simulink model "MotorIPMSVC"  (R2023a)
settings: Solver=FixedStepDiscrete  StartTime=0.0  StopTime=10.0  FixedStep=0.0001  RelTol=1e-3
InitFcn:
  | svc_go_init;
model workspace (MATLAB code in the model file):
  | cmdLim = Simulink.Parameter;
  | cmdLim.Value = 15;
  | cmdLim.Description = 'Limit for controlling the maximum surface command angle.';
  | cmdLim.Min = 0;
  | cmdLim.Max = 90;
  | cmdLim.DocUnits = 'deg';
  | 
  | dispGain = Simulink.Parameter;
  | dispGain.Value = 0.75;
  | dispGain.Description = 'Gain applied to the displacement error.';
  | dispGain.Min = 0;
  | dispGain.Max = [];
  | dispGain.DocUnits = 'deg/sec/deg';
  | 
  | dispLim = Simulink.Parameter;
  | dispLim.Value = 30;
  | dispLim.Description = 'Limit for controlling the maximum commanded angle.';
  | dispLim.Min = 0;
  | dispLim.Max = 180;
  | dispLim.DocUnits = 'deg';
  | 
  | intGain = Simulink.Parameter;
  | intGain.Value = 0.5;
  | intGain.Description = 'Gain applied to the integral error.';
  | intGain.Min = 0;
  | intGain.Max = [];
  | intGain.DocUnits = 'deg/sec/deg/sec';
  | 
  | intLim = Simulink.Parameter;
  | intLim.Value = 5;
  | intLim.Description = 'Limit for controlling the maximum commanded angle.';
  | intLim.Min = 0;
  | intLim.Max = 90;
  | intLim.DocUnits = 'deg';
  | 
  | rateGain = Simulink.Parameter;
  | rateGain.Value = 2;
  | rateGain.Description = 'Gain applied to the rate error.';
  | rateGain.Min = 0;
  | rateGain.Max = [];
  | rateGain.DocUnits = 'deg/deg/sec';
  | 
  | rateLim = Simulink.Parameter;
  | rateLim.Value = 6;
  | rateLim.Description = 'Limit for controlling the maximum commanded angle.';
  | rateLim.Min = 0;
  | rateLim.Max = 180;
  | rateLim.DocUnits = 'deg/sec';
  | 
  | hdgGain = Simulink.Parameter;
  | hdgGain.Value = 0.015;
values from neighbouring files (symbols this model uses):
  ki = 2.96*Rs/sqrt(2)/N/Ts    [svc_go_init.m]
  kp = abs(300*Ld/NTs - Rs)    [svc_go_init.m]
  Ld = 0.00026    [svc_go_init.m]
  Lq = 0.00053*(1+0.2)    (= 0.000636)    [svc_go_init.m]
  phi_r = 0.078    [svc_go_init.m]
  Rs = 0.021*(1-0.0)    (= 0.021)    [svc_go_init.m]
  Rsr = 0.021    [svc_go_init.m]
  Ts = 1/8000    (= 0.000125)    [svc_go_init.m]
  We = 2*pi*fe    (= 628.318530718)    [svc_go_init.m]
undefined symbols (not defined in the file or in its folder): DiscIntNeverNeededParam
libraries: slpidlib x4
settings Model: RequirementInfo={} %GIDa_fe9045fd_0412_4b6e_8206_617cc20e6fde  Creator=洲  LastModifiedBy=洲
settings SolverCC: AutoInsertRateTranBlk=on
settings DataIOCC: SaveOutput=off  DSMLogging=off  SaveTime=off
settings OptimizationCC: DefaultParameterBehavior=Inlined  UseDivisionForNetSlopeComputation=on  GainParamInheritBuiltInType=on  UseFloatMulNetSlope=on  UseSpecifiedMinMax=on  InlineInvariantSignals=on  EnhancedBackFolding=on  PassReuseOutputArgsAs=Individual arguments  ZeroExternalMemoryAtStartup=off  ZeroInternalMemoryAtStartup=off  NoFixptDivByZeroProtection=on  EfficientFloat2IntCast=on  LifeSpan=1  OptimizeBlockOrder=speed  DifferentSizesBufferReuse=on  OptimizationCustomize=off  EfficientTunableParamExpr=on
settings DebuggingCC: AllowSymbolicDim=off  SFUnexpectedBacktrackingDiag=warning  SFNoUnconditionalDefaultTransitionDiag=warning  SFExecutionAtInitializationDiag=none  ArithmeticOperatorsInVariantConditions=warning
settings HardwareCC: ProdLongLongMode=on
settings SFSimCC: MATLABDynamicMemAlloc=off
settings RTWCC: Description=Embedded Coder  SystemTargetFile=ert.tlc  TemplateMakefile=ert_default_tmf  BuildConfiguration=Faster Runs  DataTypeReplacement=CDataTypesFixedWidth
settings CodeAppCC: ForceParamTrailComments=on  IgnoreCustomStorageClasses=off  OperatorAnnotations=on  SimulinkDataObjDesc=on  SFDataObjDesc=on  CustomSymbolStrGlobalVar=rt$N$M  CustomSymbolStrType=$N$M  CustomSymbolStrFcn=$N$M$F  CustomSymbolStrMacro=$N$M  InsertBlockDesc=on  EnableCustomComments=on  ReqsInCode=on
settings ERTTargetCC: TargetLangStandard=C99 (ISO)  UtilityFuncGeneration=Shared location  MultiwordLength=2048  GenerateSampleERTMain=on  IncludeMdlTerminateFcn=off  CombineSignalStateStructs=on  SuppressErrorStatus=on  SupportAbsoluteTime=off  SupportNonFinite=off  SupportComplex=off  InlinedParameterPlacement=NonHierarchical  ERTCustomFileTemplate=example_file_process.tlc  ERTFilePackagingFormat=CompactWithDataFile
settings ConfigComp: CovScope=ReferencedModels  CovSaveName=covdata_rollAP  CovMetricSettings=dcmtrwe  CovHTMLOptions=-sRT=1 -aTS=1 -bRG=1 -bTC=1 -hTR=1 -nFC=0 -scm=1 -bcm=1 -xEv=0  CovSaveCumulativeToWorkspaceVar=on  CovSaveSingleToWorkspaceVar=on  CovCumulativeVarName=covCumulativeData_rollAP  CovReportOnPause=off  CovExternalEMLEnable=off  CovSFcnEnable=off

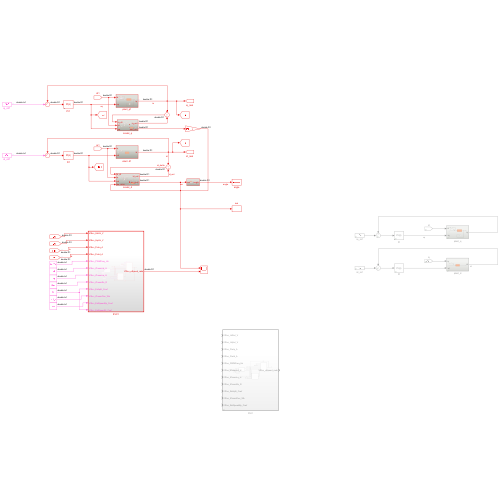
[thumbnail: Simulink's stored preview of the top-level diagram]
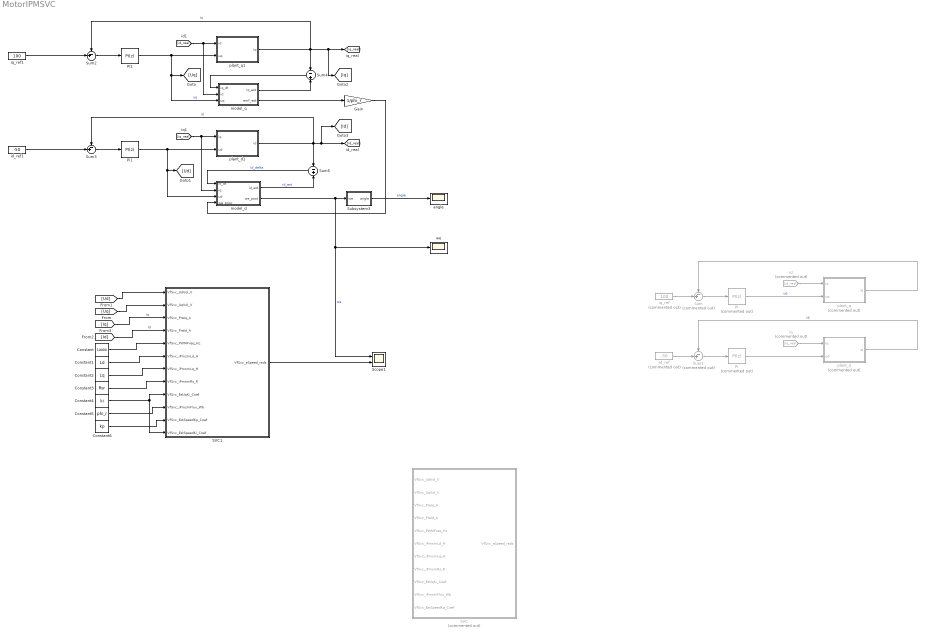
== system MotorIPMSVC ==
  Constant : Constant  Value=10000
  Constant1 : Constant  Value=Ld
  Constant2 : Constant  Value=Lq
  Constant3 : Constant  Value=Rsr
  Constant4 : Constant  Value=ki
  Constant5 : Constant  Value=phi_r
  Constant6 : Constant  Value=kp
  Gain : Gain  Gain=1/phi_r
  PI : slpidlib/PID Controller  Commented=on  Controller=PI  Form=Parallel  TimeDomain=Discrete-time  UseExternalTs=off  SampleTime=-1  IntegratorMethod=Forward Euler  FilterMethod=Forward Euler  ControllerParametersSource=internal  P=1  I=50  UseKiTs=off  D=0  N=100  UseFilter=on  TunerSelectOption=Transfer Function Based (PID Tuner App)  InitialConditionSource=internal  InitialConditionForIntegrator=0  InitialConditionForFilter=0  DifferentiatorICPrevScaledInput=0  ExternalReset=none  TrackingMode=off  Kt=1  LimitOutput=off  SatLimitsSource=internal  UpperSaturationLimit=inf  LowerSaturationLimit=-inf  LinearizeAsGain=on  AntiWindupMode=none  Kb=1  LimitIntegrator=off  UpperIntegratorSaturationLimit=inf  LowerIntegratorSaturationLimit=-inf  POutMin=[]  POutMax=[]  IOutMin=[]  IOutMax=[]  DOutMin=[]  DOutMax=[]  NOutMin=[]  NOutMax=[]  SumOutMin=[]  SumOutMax=[]  SaturationOutMin=[]  SaturationOutMax=[]  PParamMin=[]  PParamMax=[]  IParamMin=[]  IParamMax=[]  DParamMin=[]  DParamMax=[]  NParamMin=[]  NParamMax=[]  KbParamMin=[]  KbParamMax=[]  KtParamMin=[]  KtParamMax=[]  KbOutMin=[]  KbOutMax=[]  KtOutMin=[]  KtOutMax=[]  IntegratorOutMin=[]  IntegratorOutMax=[]  FilterOutMin=[]  FilterOutMax=[]  SumI1OutMin=[]  SumI1OutMax=[]  SumI2OutMin=[]  SumI2OutMax=[]  SumI3OutMin=[]  SumI3OutMax=[]  SumI4OutMin=[]  SumI4OutMax=[]  SumDOutMin=[]  SumDOutMax=[]  DifferentiatorOutMin=[]  DifferentiatorOutMax=[]  FilterDiffOutCoefMin=[]  FilterDiffOutCoefMax=[]  ReciprocalOutMin=[]  ReciprocalOutMax=[]  SumDenOutMin=[]  SumDenOutMax=[]  SumNumOutMin=[]  SumNumOutMax=[]  DivideOutMin=[]  DivideOutMax=[]  UdiffTsProdOutMin=[]  UdiffTsProdOutMax=[]  NTsProdOutMin=[]  NTsProdOutMax=[]  UintegralTsProdOutMin=[]  UintegralTsProdOutMax=[]  UngainTsProdOutMin=[]  UngainTsProdOutMax=[]  ClampingZeroOutDataTypeStr=Inherit: Inherit via back propagation  ClampingZeroOutMin=[]  ClampingZeroOutMax=[]  FilterDenConstantOutDataTypeStr=Inherit: Inherit via back propagation  FilterDenConstantOutMin=[]  FilterDenConstantOutMax=[]  PCopyOutDataTypeStr=Inherit: Inherit via back propagation  PCopyOutMin=[]  PCopyOutMax=[]  NCopyOutDataTypeStr=Inherit: Inherit via back propagation  NCopyOutMin=[]  NCopyOutMax=[]  IntegratorContinuousStateAttributes=''  IntegratorStateMustResolveToSignalObject=off  IntegratorRTWStateStorageClass=Auto  FilterContinuousStateAttributes=''  FilterStateMustResolveToSignalObject=off  FilterRTWStateStorageClass=Auto  ParallelPVariant=InternalParameters  IdealPVariant=Disabled  IVariant=InternalParameters  DVariant=Disabled  IntegratorVariant=Discrete  SatVariant=Disabled  AWVariant=Passthrough  PCopyVariant=Disabled  TRVariant=Disabled  FdbkBlocksVariant=Forward  IdealPFdbkVariant=Disabled  SatFdbkVariant=Disabled  DerivativeFilterVariant=Disabled  NVariant=Disabled  NCopyVariant=Disabled_SignalSpec  FilterICVariant=Disabled  IntegratorICVariant=InternalICs  ExternalResetVariant=Disabled  TRSumVariant=Passthrough  SumFdbkVariant=Disabled  SumVariant=Sum_PI  TsampFilterVariant=InternalTs  TsampNgainVariant=Passthrough  TsampIntegralVariant=Disabled_SignalSpec  ExternalSaturationOutDataTypeStr=Inherit: Same as second input
  PI1 : slpidlib/PID Controller  Controller=PI  Form=Parallel  TimeDomain=Discrete-time  UseExternalTs=off  SampleTime=-1  IntegratorMethod=Forward Euler  FilterMethod=Forward Euler  ControllerParametersSource=internal  P=1  I=50  UseKiTs=off  D=0  N=100  UseFilter=on  TunerSelectOption=Transfer Function Based (PID Tuner App)  InitialConditionSource=internal  InitialConditionForIntegrator=0  InitialConditionForFilter=0  DifferentiatorICPrevScaledInput=0  ExternalReset=none  TrackingMode=off  Kt=1  LimitOutput=off  SatLimitsSource=internal  UpperSaturationLimit=inf  LowerSaturationLimit=-inf  LinearizeAsGain=on  AntiWindupMode=none  Kb=1  LimitIntegrator=off  UpperIntegratorSaturationLimit=inf  LowerIntegratorSaturationLimit=-inf  POutMin=[]  POutMax=[]  IOutMin=[]  IOutMax=[]  DOutMin=[]  DOutMax=[]  NOutMin=[]  NOutMax=[]  SumOutMin=[]  SumOutMax=[]  SaturationOutMin=[]  SaturationOutMax=[]  PParamMin=[]  PParamMax=[]  IParamMin=[]  IParamMax=[]  DParamMin=[]  DParamMax=[]  NParamMin=[]  NParamMax=[]  KbParamMin=[]  KbParamMax=[]  KtParamMin=[]  KtParamMax=[]  KbOutMin=[]  KbOutMax=[]  KtOutMin=[]  KtOutMax=[]  IntegratorOutMin=[]  IntegratorOutMax=[]  FilterOutMin=[]  FilterOutMax=[]  SumI1OutMin=[]  SumI1OutMax=[]  SumI2OutMin=[]  SumI2OutMax=[]  SumI3OutMin=[]  SumI3OutMax=[]  SumI4OutMin=[]  SumI4OutMax=[]  SumDOutMin=[]  SumDOutMax=[]  DifferentiatorOutMin=[]  DifferentiatorOutMax=[]  FilterDiffOutCoefMin=[]  FilterDiffOutCoefMax=[]  ReciprocalOutMin=[]  ReciprocalOutMax=[]  SumDenOutMin=[]  SumDenOutMax=[]  SumNumOutMin=[]  SumNumOutMax=[]  DivideOutMin=[]  DivideOutMax=[]  UdiffTsProdOutMin=[]  UdiffTsProdOutMax=[]  NTsProdOutMin=[]  NTsProdOutMax=[]  UintegralTsProdOutMin=[]  UintegralTsProdOutMax=[]  UngainTsProdOutMin=[]  UngainTsProdOutMax=[]  ClampingZeroOutDataTypeStr=Inherit: Inherit via back propagation  ClampingZeroOutMin=[]  ClampingZeroOutMax=[]  FilterDenConstantOutDataTypeStr=Inherit: Inherit via back propagation  FilterDenConstantOutMin=[]  FilterDenConstantOutMax=[]  PCopyOutDataTypeStr=Inherit: Inherit via back propagation  PCopyOutMin=[]  PCopyOutMax=[]  NCopyOutDataTypeStr=Inherit: Inherit via back propagation  NCopyOutMin=[]  NCopyOutMax=[]  IntegratorContinuousStateAttributes=''  IntegratorStateMustResolveToSignalObject=off  IntegratorRTWStateStorageClass=Auto  FilterContinuousStateAttributes=''  FilterStateMustResolveToSignalObject=off  FilterRTWStateStorageClass=Auto  ParallelPVariant=InternalParameters  IdealPVariant=Disabled  IVariant=InternalParameters  DVariant=Disabled  IntegratorVariant=Discrete  SatVariant=Disabled  AWVariant=Passthrough  PCopyVariant=Disabled  TRVariant=Disabled  FdbkBlocksVariant=Forward  IdealPFdbkVariant=Disabled  SatFdbkVariant=Disabled  DerivativeFilterVariant=Disabled  NVariant=Disabled  NCopyVariant=Disabled_SignalSpec  FilterICVariant=Disabled  IntegratorICVariant=InternalICs  ExternalResetVariant=Disabled  TRSumVariant=Passthrough  SumFdbkVariant=Disabled  SumVariant=Sum_PI  TsampFilterVariant=InternalTs  TsampNgainVariant=Passthrough  TsampIntegralVariant=Disabled_SignalSpec  ExternalSaturationOutDataTypeStr=Inherit: Same as second input
  Pi : slpidlib/PID Controller  Commented=on  Controller=PI  Form=Parallel  TimeDomain=Discrete-time  UseExternalTs=off  SampleTime=-1  IntegratorMethod=Forward Euler  FilterMethod=Forward Euler  ControllerParametersSource=internal  P=1  I=50  UseKiTs=off  D=0  N=100  UseFilter=on  TunerSelectOption=Transfer Function Based (PID Tuner App)  InitialConditionSource=internal  InitialConditionForIntegrator=0  InitialConditionForFilter=0  DifferentiatorICPrevScaledInput=0  ExternalReset=none  TrackingMode=off  Kt=1  LimitOutput=off  SatLimitsSource=internal  UpperSaturationLimit=inf  LowerSaturationLimit=-inf  LinearizeAsGain=on  AntiWindupMode=none  Kb=1  LimitIntegrator=off  UpperIntegratorSaturationLimit=inf  LowerIntegratorSaturationLimit=-inf  POutMin=[]  POutMax=[]  IOutMin=[]  IOutMax=[]  DOutMin=[]  DOutMax=[]  NOutMin=[]  NOutMax=[]  SumOutMin=[]  SumOutMax=[]  SaturationOutMin=[]  SaturationOutMax=[]  PParamMin=[]  PParamMax=[]  IParamMin=[]  IParamMax=[]  DParamMin=[]  DParamMax=[]  NParamMin=[]  NParamMax=[]  KbParamMin=[]  KbParamMax=[]  KtParamMin=[]  KtParamMax=[]  KbOutMin=[]  KbOutMax=[]  KtOutMin=[]  KtOutMax=[]  IntegratorOutMin=[]  IntegratorOutMax=[]  FilterOutMin=[]  FilterOutMax=[]  SumI1OutMin=[]  SumI1OutMax=[]  SumI2OutMin=[]  SumI2OutMax=[]  SumI3OutMin=[]  SumI3OutMax=[]  SumI4OutMin=[]  SumI4OutMax=[]  SumDOutMin=[]  SumDOutMax=[]  DifferentiatorOutMin=[]  DifferentiatorOutMax=[]  FilterDiffOutCoefMin=[]  FilterDiffOutCoefMax=[]  ReciprocalOutMin=[]  ReciprocalOutMax=[]  SumDenOutMin=[]  SumDenOutMax=[]  SumNumOutMin=[]  SumNumOutMax=[]  DivideOutMin=[]  DivideOutMax=[]  UdiffTsProdOutMin=[]  UdiffTsProdOutMax=[]  NTsProdOutMin=[]  NTsProdOutMax=[]  UintegralTsProdOutMin=[]  UintegralTsProdOutMax=[]  UngainTsProdOutMin=[]  UngainTsProdOutMax=[]  ClampingZeroOutDataTypeStr=Inherit: Inherit via back propagation  ClampingZeroOutMin=[]  ClampingZeroOutMax=[]  FilterDenConstantOutDataTypeStr=Inherit: Inherit via back propagation  FilterDenConstantOutMin=[]  FilterDenConstantOutMax=[]  PCopyOutDataTypeStr=Inherit: Inherit via back propagation  PCopyOutMin=[]  PCopyOutMax=[]  NCopyOutDataTypeStr=Inherit: Inherit via back propagation  NCopyOutMin=[]  NCopyOutMax=[]  IntegratorContinuousStateAttributes=''  IntegratorStateMustResolveToSignalObject=off  IntegratorRTWStateStorageClass=Auto  FilterContinuousStateAttributes=''  FilterStateMustResolveToSignalObject=off  FilterRTWStateStorageClass=Auto  ParallelPVariant=InternalParameters  IdealPVariant=Disabled  IVariant=InternalParameters  DVariant=Disabled  IntegratorVariant=Discrete  SatVariant=Disabled  AWVariant=Passthrough  PCopyVariant=Disabled  TRVariant=Disabled  FdbkBlocksVariant=Forward  IdealPFdbkVariant=Disabled  SatFdbkVariant=Disabled  DerivativeFilterVariant=Disabled  NVariant=Disabled  NCopyVariant=Disabled_SignalSpec  FilterICVariant=Disabled  IntegratorICVariant=InternalICs  ExternalResetVariant=Disabled  TRSumVariant=Passthrough  SumFdbkVariant=Disabled  SumVariant=Sum_PI  TsampFilterVariant=InternalTs  TsampNgainVariant=Passthrough  TsampIntegralVariant=Disabled_SignalSpec  ExternalSaturationOutDataTypeStr=Inherit: Same as second input
  Pi1 : slpidlib/PID Controller  Controller=PI  Form=Parallel  TimeDomain=Discrete-time  UseExternalTs=off  SampleTime=-1  IntegratorMethod=Forward Euler  FilterMethod=Forward Euler  ControllerParametersSource=internal  P=1  I=50  UseKiTs=off  D=0  N=100  UseFilter=on  TunerSelectOption=Transfer Function Based (PID Tuner App)  InitialConditionSource=internal  InitialConditionForIntegrator=0  InitialConditionForFilter=0  DifferentiatorICPrevScaledInput=0  ExternalReset=none  TrackingMode=off  Kt=1  LimitOutput=off  SatLimitsSource=internal  UpperSaturationLimit=inf  LowerSaturationLimit=-inf  LinearizeAsGain=on  AntiWindupMode=none  Kb=1  LimitIntegrator=off  UpperIntegratorSaturationLimit=inf  LowerIntegratorSaturationLimit=-inf  POutMin=[]  POutMax=[]  IOutMin=[]  IOutMax=[]  DOutMin=[]  DOutMax=[]  NOutMin=[]  NOutMax=[]  SumOutMin=[]  SumOutMax=[]  SaturationOutMin=[]  SaturationOutMax=[]  PParamMin=[]  PParamMax=[]  IParamMin=[]  IParamMax=[]  DParamMin=[]  DParamMax=[]  NParamMin=[]  NParamMax=[]  KbParamMin=[]  KbParamMax=[]  KtParamMin=[]  KtParamMax=[]  KbOutMin=[]  KbOutMax=[]  KtOutMin=[]  KtOutMax=[]  IntegratorOutMin=[]  IntegratorOutMax=[]  FilterOutMin=[]  FilterOutMax=[]  SumI1OutMin=[]  SumI1OutMax=[]  SumI2OutMin=[]  SumI2OutMax=[]  SumI3OutMin=[]  SumI3OutMax=[]  SumI4OutMin=[]  SumI4OutMax=[]  SumDOutMin=[]  SumDOutMax=[]  DifferentiatorOutMin=[]  DifferentiatorOutMax=[]  FilterDiffOutCoefMin=[]  FilterDiffOutCoefMax=[]  ReciprocalOutMin=[]  ReciprocalOutMax=[]  SumDenOutMin=[]  SumDenOutMax=[]  SumNumOutMin=[]  SumNumOutMax=[]  DivideOutMin=[]  DivideOutMax=[]  UdiffTsProdOutMin=[]  UdiffTsProdOutMax=[]  NTsProdOutMin=[]  NTsProdOutMax=[]  UintegralTsProdOutMin=[]  UintegralTsProdOutMax=[]  UngainTsProdOutMin=[]  UngainTsProdOutMax=[]  ClampingZeroOutDataTypeStr=Inherit: Inherit via back propagation  ClampingZeroOutMin=[]  ClampingZeroOutMax=[]  FilterDenConstantOutDataTypeStr=Inherit: Inherit via back propagation  FilterDenConstantOutMin=[]  FilterDenConstantOutMax=[]  PCopyOutDataTypeStr=Inherit: Inherit via back propagation  PCopyOutMin=[]  PCopyOutMax=[]  NCopyOutDataTypeStr=Inherit: Inherit via back propagation  NCopyOutMin=[]  NCopyOutMax=[]  IntegratorContinuousStateAttributes=''  IntegratorStateMustResolveToSignalObject=off  IntegratorRTWStateStorageClass=Auto  FilterContinuousStateAttributes=''  FilterStateMustResolveToSignalObject=off  FilterRTWStateStorageClass=Auto  ParallelPVariant=InternalParameters  IdealPVariant=Disabled  IVariant=InternalParameters  DVariant=Disabled  IntegratorVariant=Discrete  SatVariant=Disabled  AWVariant=Passthrough  PCopyVariant=Disabled  TRVariant=Disabled  FdbkBlocksVariant=Forward  IdealPFdbkVariant=Disabled  SatFdbkVariant=Disabled  DerivativeFilterVariant=Disabled  NVariant=Disabled  NCopyVariant=Disabled_SignalSpec  FilterICVariant=Disabled  IntegratorICVariant=InternalICs  ExternalResetVariant=Disabled  TRSumVariant=Passthrough  SumFdbkVariant=Disabled  SumVariant=Sum_PI  TsampFilterVariant=InternalTs  TsampNgainVariant=Passthrough  TsampIntegralVariant=Disabled_SignalSpec  ExternalSaturationOutDataTypeStr=Inherit: Same as second input
  SVC : Subsystem  Commented=on  TreatAsAtomicUnit=on
      settings: RTWSystemCode=Nonreusable function
  SVC1 : Subsystem  TreatAsAtomicUnit=on
      settings: RTWSystemCode=Nonreusable function
  Scope1 : Scope  NumInputPorts=2
  Subsystem3 : Subsystem
  Sum : Sum  Commented=on  Inputs=-+|
  Sum1 : Sum  Commented=on  Inputs=-+|
  Sum2 : Sum  Inputs=-+|
  Sum3 : Sum  Inputs=-+|
  Sum4 : Sum  Inputs=-+
  Sum5 : Sum  Inputs=-+
  angle : Scope
  id : From  Commented=on  GotoTag=id_real
  id_ref : Constant  Commented=on  Value=-50
  id_ref1 : Constant  Value=-50
  iq : From  Commented=on  GotoTag=iq_real
  iq_ref : Constant  Commented=on  Value=100
  iq_ref1 : Constant  Value=100
  model_d : Subsystem
  model_q : Subsystem
  plant_d : Subsystem  Commented=on
  plant_d1 : Subsystem
  plant_q : Subsystem  Commented=on
  plant_q1 : Subsystem
  we : Scope
  wires:
  plant_q/1(iq) -> Sum/1
  id/1 -> plant_q/1(id)
  PI/1 -> plant_q/2(uq)  "uq"
  Sum/1 -> PI/1
  iq_ref/1 -> Sum/2
  iq/1 -> plant_d/1(iq)
  Sum1/1 -> Pi/1
  plant_d/1(id) -> Sum1/1  "id"
  Pi/1 -> plant_d/2(ud)
  id_ref/1 -> Sum1/2
  [Uq] -> SVC1/2(VfSvc_UqVol_V)
  [Ud] -> SVC1/1(VfSvc_UdVol_V)
  [Iq] -> SVC1/3(VfSvc_PreIq_A)  "Iq"
  [Id] -> SVC1/4(VfSvc_PreId_A)  "Id"
  Constant/1 -> SVC1/5(VfSvc_PWMFreq_Hz)
  Constant1/1 -> SVC1/6(VfSvc_iPmsmLd_H)
  Constant2/1 -> SVC1/7(VfSvc_iPmsmLq_H)
  Constant3/1 -> SVC1/8(VfSvc_iPmsmRs_R)
  Constant4/1 -> SVC1/12(VfSvc_EstSpeedKi_Coef), SVC1/9(VfSvc_EstIqKi_Coef)
  Constant5/1 -> SVC1/10(VfSvc_iPmsmFlux_Wb)
  Constant6/1 -> SVC1/11(VfSvc_EstSpeedKp_Coef)
  SVC1/1(VfSvc_eSpeed_rads) -> Scope1/2
  [iq_real] -> plant_d1/1(iq), model_d/2(iq)
  model_q/2(emf_est) -> Gain/1
  model_d/1(id_est) -> Sum5/2  "id_est"
  Sum3/1 -> Pi1/1
  plant_d1/1(id) -> Sum3/1, Sum5/1, [Id], [id_real]  "id"
  Pi1/1 -> [Ud], model_d/3(ud), plant_d1/2(ud)
  Sum5/1 -> model_d/1(id_dt)  "id_delta"
  model_q/1(iq_est) -> Sum4/2
  [id_real] -> model_q/2(id), plant_q1/1(id)
  PI1/1 -> plant_q1/2(uq), model_q/3(uq), [Uq]  "uq"
  Sum2/1 -> PI1/1
  Gain/1 -> model_d/4(we_prior)
  Subsystem3/1(angle) -> angle/1  "angle"
  iq_ref1/1 -> Sum2/2
  id_ref1/1 -> Sum3/2
  model_d/2(we_post) -> Scope1/1, we/1, Subsystem3/1(we)  "we"
  Sum4/1 -> model_q/1(iq_dt)
  plant_q1/1(iq) -> Sum2/1, [Iq], [iq_real], Sum4/1  "iq"

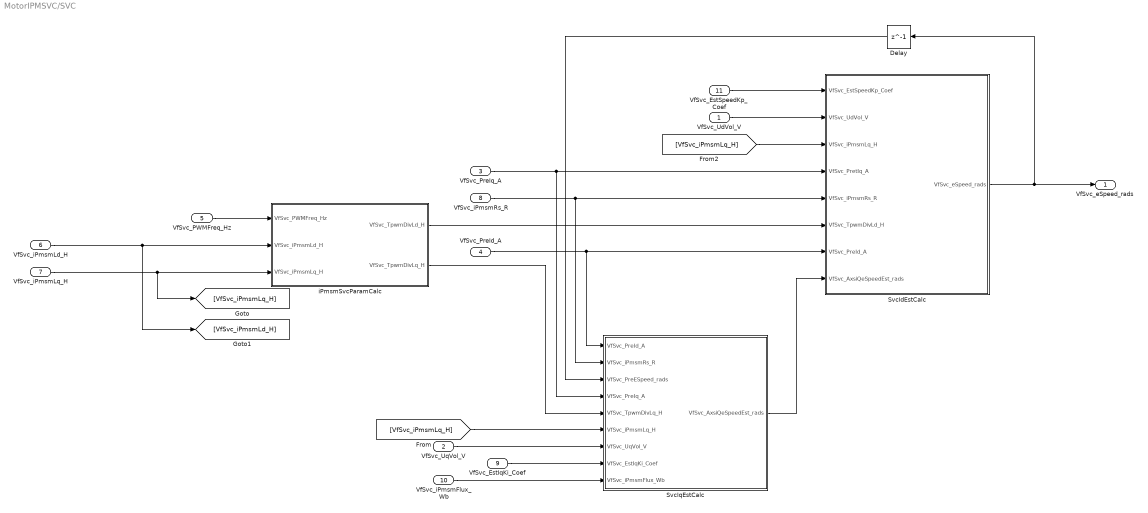
== system MotorIPMSVC/SVC ==
  VfSvc_UdVol_V : Inport
  VfSvc_UqVol_V : Inport  Port=2
  VfSvc_PreIq_A : Inport  Port=3
  VfSvc_PreId_A : Inport  Port=4
  VfSvc_PWMFreq_Hz : Inport  Port=5
  VfSvc_iPmsmLd_H : Inport  Port=6
  VfSvc_iPmsmLq_H : Inport  Port=7
  VfSvc_iPmsmRs_R : Inport  Port=8
  VfSvc_EstIqKi_Coef : Inport  Port=9
  VfSvc_iPmsmFlux_Wb : Inport  Port=10
  VfSvc_EstSpeedKp_Coef : Inport  Port=11
  Delay : Delay  DelayLength=1
  SvcIdEstCalc : Subsystem
  SvcIqEstCalc : Subsystem
  iPmsmSvcParamCalc : Subsystem  TreatAsAtomicUnit=on
      settings: RTWSystemCode=Nonreusable function  RTWFcnNameOpts=Use subsystem name
  VfSvc_eSpeed_rads : Outport
  wires:
  iPmsmSvcParamCalc/1(VfSvc_TpwmDivLd_H) -> SvcIdEstCalc/6(VfSvc_TpwmDivLd_H)
  SvcIqEstCalc/1(VfSvc_AxsiQeSpeedEst_rads) -> SvcIdEstCalc/8(VfSvc_AxsiQeSpeedEst_rads)
  VfSvc_iPmsmLq_H/1 -> iPmsmSvcParamCalc/3(VfSvc_iPmsmLq_H), [VfSvc_iPmsmLq_H]
  VfSvc_PreIq_A/1 -> SvcIqEstCalc/4(VfSvc_PreIq_A), SvcIdEstCalc/4(VfSvc_PretIq_A)
  VfSvc_iPmsmFlux_Wb/1 -> SvcIqEstCalc/9(VfSvc_iPmsmFlux_Wb)
  VfSvc_iPmsmRs_R/1 -> SvcIqEstCalc/2(VfSvc_iPmsmRs_R), SvcIdEstCalc/5(VfSvc_iPmsmRs_R)
  VfSvc_PWMFreq_Hz/1 -> iPmsmSvcParamCalc/1(VfSvc_PWMFreq_Hz)
  SvcIdEstCalc/1(VfSvc_eSpeed_rads) -> VfSvc_eSpeed_rads/1, Delay/1
  iPmsmSvcParamCalc/2(VfSvc_TpwmDivLq_H) -> SvcIqEstCalc/5(VfSvc_TpwmDivLq_H)
  VfSvc_PreId_A/1 -> SvcIqEstCalc/1(VfSvc_PreId_A), SvcIdEstCalc/7(VfSvc_PreId_A)
  VfSvc_iPmsmLd_H/1 -> [VfSvc_iPmsmLd_H], iPmsmSvcParamCalc/2(VfSvc_iPmsmLd_H)
  VfSvc_UdVol_V/1 -> SvcIdEstCalc/2(VfSvc_UdVol_V)
  VfSvc_UqVol_V/1 -> SvcIqEstCalc/7(VfSvc_UqVol_V)
  [VfSvc_iPmsmLq_H] -> SvcIqEstCalc/6(VfSvc_iPmsmLq_H)
  VfSvc_EstIqKi_Coef/1 -> SvcIqEstCalc/8(VfSvc_EstIqKi_Coef)
  VfSvc_EstSpeedKp_Coef/1 -> SvcIdEstCalc/1(VfSvc_EstSpeedKp_Coef)
  Delay/1 -> SvcIqEstCalc/3(VfSvc_PreESpeed_rads)
  [VfSvc_iPmsmLq_H] -> SvcIdEstCalc/3(VfSvc_iPmsmLq_H)

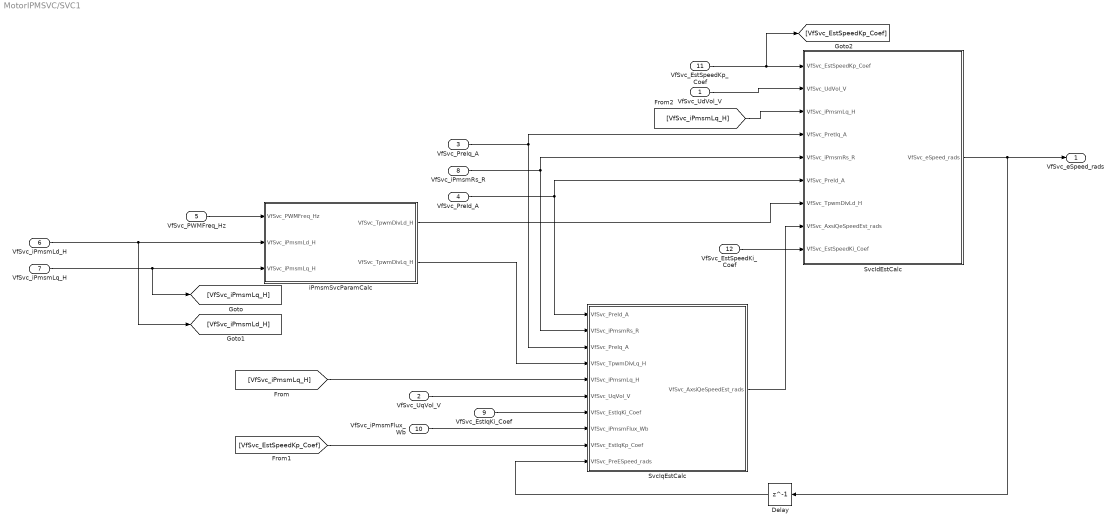
== system MotorIPMSVC/SVC1 ==
  VfSvc_UdVol_V : Inport
  VfSvc_UqVol_V : Inport  Port=2
  VfSvc_PreIq_A : Inport  Port=3
  VfSvc_PreId_A : Inport  Port=4
  VfSvc_PWMFreq_Hz : Inport  Port=5
  VfSvc_iPmsmLd_H : Inport  Port=6
  VfSvc_iPmsmLq_H : Inport  Port=7
  VfSvc_iPmsmRs_R : Inport  Port=8
  VfSvc_EstIqKi_Coef : Inport  Port=9
  VfSvc_iPmsmFlux_Wb : Inport  Port=10
  VfSvc_EstSpeedKp_Coef : Inport  Port=11
  VfSvc_EstSpeedKi_Coef : Inport  Port=12
  Delay : Delay  DelayLength=1
  SvcIdEstCalc : Subsystem
  SvcIqEstCalc : Subsystem  TreatAsAtomicUnit=on
      settings: RTWSystemCode=Nonreusable function
  iPmsmSvcParamCalc : Subsystem  TreatAsAtomicUnit=on
      settings: RTWSystemCode=Nonreusable function  RTWFcnNameOpts=Use subsystem name
  VfSvc_eSpeed_rads : Outport
  wires:
  iPmsmSvcParamCalc/1(VfSvc_TpwmDivLd_H) -> SvcIdEstCalc/7(VfSvc_TpwmDivLd_H)
  SvcIqEstCalc/1(VfSvc_AxsiQeSpeedEst_rads) -> SvcIdEstCalc/8(VfSvc_AxsiQeSpeedEst_rads)
  VfSvc_iPmsmLq_H/1 -> iPmsmSvcParamCalc/3(VfSvc_iPmsmLq_H), [VfSvc_iPmsmLq_H]
  VfSvc_PreIq_A/1 -> SvcIdEstCalc/4(VfSvc_PretIq_A), SvcIqEstCalc/3(VfSvc_PreIq_A)
  VfSvc_iPmsmFlux_Wb/1 -> SvcIqEstCalc/8(VfSvc_iPmsmFlux_Wb)
  VfSvc_iPmsmRs_R/1 -> SvcIdEstCalc/5(VfSvc_iPmsmRs_R), SvcIqEstCalc/2(VfSvc_iPmsmRs_R)
  VfSvc_PWMFreq_Hz/1 -> iPmsmSvcParamCalc/1(VfSvc_PWMFreq_Hz)
  SvcIdEstCalc/1(VfSvc_eSpeed_rads) -> Delay/1, VfSvc_eSpeed_rads/1
  iPmsmSvcParamCalc/2(VfSvc_TpwmDivLq_H) -> SvcIqEstCalc/4(VfSvc_TpwmDivLq_H)
  VfSvc_PreId_A/1 -> SvcIqEstCalc/1(VfSvc_PreId_A), SvcIdEstCalc/6(VfSvc_PreId_A)
  VfSvc_iPmsmLd_H/1 -> [VfSvc_iPmsmLd_H], iPmsmSvcParamCalc/2(VfSvc_iPmsmLd_H)
  VfSvc_UdVol_V/1 -> SvcIdEstCalc/2(VfSvc_UdVol_V)
  VfSvc_UqVol_V/1 -> SvcIqEstCalc/6(VfSvc_UqVol_V)
  [VfSvc_iPmsmLq_H] -> SvcIqEstCalc/5(VfSvc_iPmsmLq_H)
  VfSvc_EstIqKi_Coef/1 -> SvcIqEstCalc/7(VfSvc_EstIqKi_Coef)
  VfSvc_EstSpeedKp_Coef/1 -> [VfSvc_EstSpeedKp_Coef], SvcIdEstCalc/1(VfSvc_EstSpeedKp_Coef)
  Delay/1 -> SvcIqEstCalc/10(VfSvc_PreESpeed_rads)
  [VfSvc_iPmsmLq_H] -> SvcIdEstCalc/3(VfSvc_iPmsmLq_H)
  [VfSvc_EstSpeedKp_Coef] -> SvcIqEstCalc/9(VfSvc_EstIqKp_Coef)
  VfSvc_EstSpeedKi_Coef/1 -> SvcIdEstCalc/9(VfSvc_EstSpeedKi_Coef)

== system MotorIPMSVC/Subsystem3 ==
  we : Inport
  Constant : Constant  Value=2*pi
  Discrete-Time Integrator : DiscreteIntegrator  SampleTime=-1  ICPrevOutput=DiscIntNeverNeededParam  ICPrevScaledInput=DiscIntNeverNeededParam
  Mod : Math  Operator=mod  SignedPower=on
  angle : Outport  VectorParamsAs1DForOutWhenUnconnected=off
  wires:
  Constant/1 -> Mod/2
  we/1 -> Discrete-Time Integrator/1
  Mod/1 -> angle/1
  Discrete-Time Integrator/1 -> Mod/1  "angle"

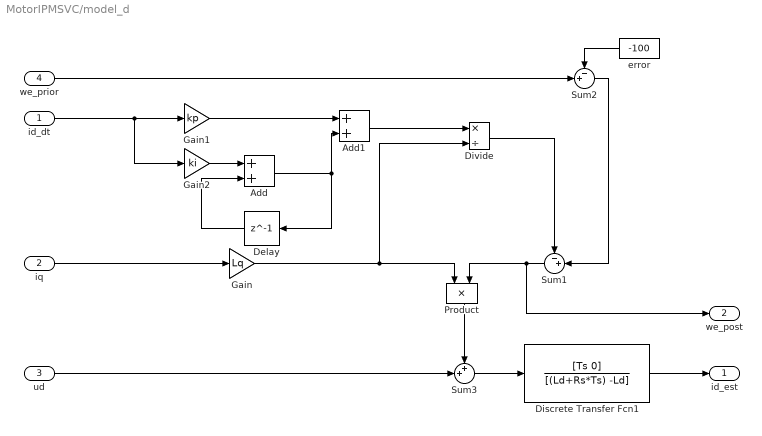
== system MotorIPMSVC/model_d ==
  id_dt : Inport
  iq : Inport  Port=2
  ud : Inport  Port=3
  we_prior : Inport  Port=4
  Add : Sum
  Add1 : Sum
  Delay : Delay  DelayLength=1
  Discrete Transfer Fcn1 : DiscreteTransferFcn  Numerator=[Ts 0]  Denominator=[(Ld+Rs*Ts) -Ld]
  Divide : Product  Inputs=*/
  Gain : Gain  Gain=Lq
  Gain1 : Gain  Gain=kp
  Gain2 : Gain  Gain=ki
  Product : Product
  Sum1 : Sum  Inputs=-+|
  Sum2 : Sum  Inputs=-+|
  Sum3 : Sum  Inputs=++|
  error : Constant  Value=-100
  id_est : Outport  VectorParamsAs1DForOutWhenUnconnected=off
  we_post : Outport  Port=2  VectorParamsAs1DForOutWhenUnconnected=off
  wires:
  iq/1 -> Gain/1
  ud/1 -> Sum3/2
  Sum3/1 -> Discrete Transfer Fcn1/1
  Gain/1 -> Product/1, Divide/2
  Product/1 -> Sum3/1
  Sum1/1 -> Product/2, we_post/1
  we_prior/1 -> Sum2/2
  error/1 -> Sum2/1
  Sum2/1 -> Sum1/2
  Discrete Transfer Fcn1/1 -> id_est/1
  id_dt/1 -> Gain2/1, Gain1/1
  Divide/1 -> Sum1/1
  Gain1/1 -> Add1/1
  Gain2/1 -> Add/1
  Add/1 -> Delay/1, Add1/2
  Delay/1 -> Add/2
  Add1/1 -> Divide/1

== system MotorIPMSVC/model_q ==
  iq_dt : Inport
  id : Inport  Port=2
  uq : Inport  Port=3
  Add : Sum
  Add1 : Sum
  Delay : Delay  DelayLength=1
  Discrete Transfer Fcn2 : DiscreteTransferFcn  Numerator=[Ts 0]  Denominator=[(Lq+Rs*Ts) -Lq]
  Gain : Gain  Gain=We*Ld
  Gain1 : Gain  Gain=kp
  Gain2 : Gain  Gain=ki
  Sum : Sum  Inputs=--+|
  iq_est : Outport  VectorParamsAs1DForOutWhenUnconnected=off
  emf_est : Outport  Port=2  VectorParamsAs1DForOutWhenUnconnected=off
  wires:
  iq_dt/1 -> Gain1/1, Gain2/1  "est"
  Gain/1 -> Sum/2
  uq/1 -> Sum/3
  Sum/1 -> Discrete Transfer Fcn2/1
  Add1/1 -> emf_est/1, Sum/1
  Discrete Transfer Fcn2/1 -> iq_est/1  "iq"
  id/1 -> Gain/1
  Delay/1 -> Add/2
  Gain1/1 -> Add1/1
  Gain2/1 -> Add/1
  Add/1 -> Delay/1, Add1/2

== system MotorIPMSVC/plant_d ==
  iq : Inport
  ud : Inport  Port=2
  Discrete Transfer Fcn1 : DiscreteTransferFcn  Numerator=[Ts 0]  Denominator=[(Ld+Rs*Ts) -Ld]
  Gain : Gain  Gain=We*Lq
  Sum3 : Sum  Inputs=++|
  id : Outport  VectorParamsAs1DForOutWhenUnconnected=off
  wires:
  iq/1 -> Gain/1
  ud/1 -> Sum3/2
  Sum3/1 -> Discrete Transfer Fcn1/1
  Gain/1 -> Sum3/1
  Discrete Transfer Fcn1/1 -> id/1

== system MotorIPMSVC/plant_d1 ==
  iq : Inport
  ud : Inport  Port=2
  Discrete Transfer Fcn1 : DiscreteTransferFcn  Numerator=[Ts 0]  Denominator=[(Ld+Rs*Ts) -Ld]
  Gain : Gain  Gain=We*Lq
  Sum3 : Sum  Inputs=++|
  id : Outport  VectorParamsAs1DForOutWhenUnconnected=off
  wires:
  iq/1 -> Gain/1
  ud/1 -> Sum3/2
  Sum3/1 -> Discrete Transfer Fcn1/1
  Gain/1 -> Sum3/1
  Discrete Transfer Fcn1/1 -> id/1

== system MotorIPMSVC/plant_q ==
  id : Inport
  uq : Inport  Port=2
  Constant : Constant  Value=We*phi_r
  Discrete Transfer Fcn1 : DiscreteTransferFcn  Numerator=[Ts 0]  Denominator=[(Lq+Rs*Ts) -Lq]
  Gain : Gain  Gain=We*Ld
  Sum : Sum  Inputs=--+|
  we1 : Scope  NumInputPorts=2
  iq : Outport  VectorParamsAs1DForOutWhenUnconnected=off
  wires:
  id/1 -> Gain/1
  Discrete Transfer Fcn1/1 -> we1/1, iq/1  "iq"
  Sum/1 -> Discrete Transfer Fcn1/1
  uq/1 -> Sum/3
  Gain/1 -> Sum/1
  Constant/1 -> Sum/2

== system MotorIPMSVC/plant_q1 ==
  id : Inport
  uq : Inport  Port=2
  Constant : Constant  Value=We*phi_r
  Discrete Transfer Fcn1 : DiscreteTransferFcn  Numerator=[Ts 0]  Denominator=[(Lq+Rs*Ts) -Lq]
  Gain : Gain  Gain=We*Ld
  Sum : Sum  Inputs=--+|
  we1 : Scope  NumInputPorts=2
  iq : Outport  VectorParamsAs1DForOutWhenUnconnected=off
  wires:
  id/1 -> Gain/1
  Discrete Transfer Fcn1/1 -> we1/1, iq/1  "iq"
  Sum/1 -> Discrete Transfer Fcn1/1
  uq/1 -> Sum/3
  Gain/1 -> Sum/1
  Constant/1 -> Sum/2

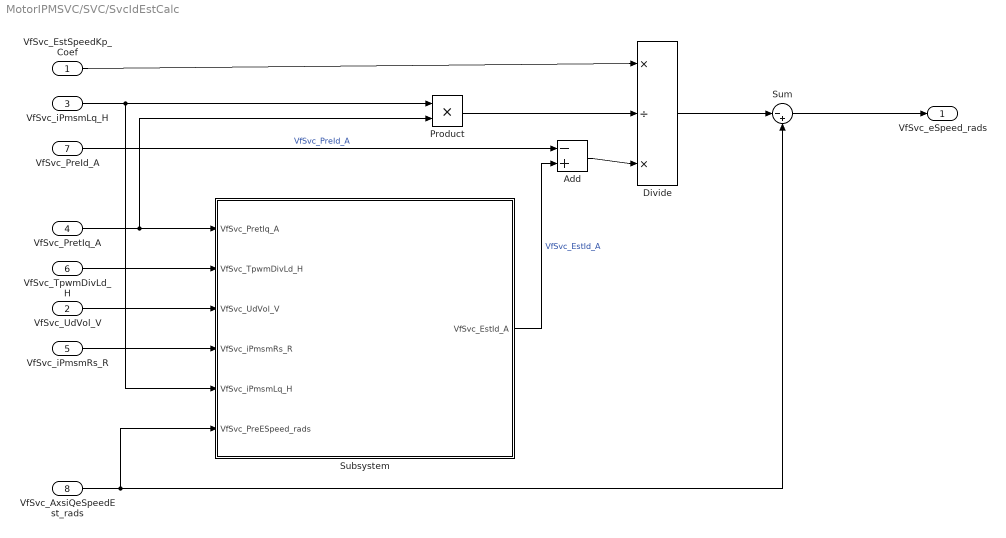
== system MotorIPMSVC/SVC/SvcIdEstCalc ==
  VfSvc_EstSpeedKp_Coef : Inport
  VfSvc_UdVol_V : Inport  Port=2
  VfSvc_iPmsmLq_H : Inport  Port=3
  VfSvc_PretIq_A : Inport  Port=4
  VfSvc_iPmsmRs_R : Inport  Port=5
  VfSvc_TpwmDivLd_H : Inport  Port=6
  VfSvc_PreId_A : Inport  Port=7
  VfSvc_AxsiQeSpeedEst_rads : Inport  Port=8
  Add : Sum  Inputs=-+
  Divide : Product  Inputs=*/*
  Product : Product
  Subsystem : Subsystem
  Sum : Sum  Inputs=|-+
  VfSvc_eSpeed_rads : Outport
  wires:
  VfSvc_TpwmDivLd_H/1 -> Subsystem/2(VfSvc_TpwmDivLd_H)
  VfSvc_UdVol_V/1 -> Subsystem/3(VfSvc_UdVol_V)
  VfSvc_PretIq_A/1 -> Product/2, Subsystem/1(VfSvc_PretIq_A)
  VfSvc_iPmsmRs_R/1 -> Subsystem/4(VfSvc_iPmsmRs_R)
  VfSvc_iPmsmLq_H/1 -> Subsystem/5(VfSvc_iPmsmLq_H), Product/1
  Subsystem/1(VfSvc_EstId_A) -> Add/2  "VfSvc_EstId_A"
  VfSvc_EstSpeedKp_Coef/1 -> Divide/1
  Add/1 -> Divide/3
  VfSvc_PreId_A/1 -> Add/1  "VfSvc_PreId_A"
  VfSvc_AxsiQeSpeedEst_rads/1 -> Sum/2, Subsystem/6(VfSvc_PreESpeed_rads)
  Sum/1 -> VfSvc_eSpeed_rads/1
  Product/1 -> Divide/2
  Divide/1 -> Sum/1

== system MotorIPMSVC/SVC/SvcIqEstCalc ==
  VfSvc_PreId_A : Inport
  VfSvc_iPmsmRs_R : Inport  Port=2
  VfSvc_PreESpeed_rads : Inport  Port=3
  VfSvc_PreIq_A : Inport  Port=4
  VfSvc_TpwmDivLq_H : Inport  Port=5
  VfSvc_iPmsmLq_H : Inport  Port=6
  VfSvc_UqVol_V : Inport  Port=7
  VfSvc_EstIqKi_Coef : Inport  Port=8
  VfSvc_iPmsmFlux_Wb : Inport  Port=9
  Delay : Delay  DelayLength=1
  Subsystem : Subsystem
  Subsystem1 : Subsystem
  VfSvc_AxsiQeSpeedEst_rads : Outport
  wires:
  VfSvc_PreId_A/1 -> Subsystem/1(VfSvc_PreId_A)
  VfSvc_TpwmDivLq_H/1 -> Subsystem/2(VfSvc_TpwmDivLq_H)
  VfSvc_UqVol_V/1 -> Subsystem/3(VfSvc_UqVol_V)
  VfSvc_PreESpeed_rads/1 -> Subsystem/4(VfSvc_PreESpeed_rads)
  VfSvc_iPmsmRs_R/1 -> Subsystem/5(VfSvc_iPmsmRs_R)
  VfSvc_iPmsmLq_H/1 -> Subsystem/6(VfSvc_iPmsmLq_H)
  Subsystem/1(VfSvc_EstIq_A) -> Subsystem1/1(VfSvc_EstIq_A)  "VfSvc_EstIq_A"
  VfSvc_EstIqKi_Coef/1 -> Subsystem1/2(VfSvc_EstIqKi_Coef)
  Subsystem1/1(VfSvc_iPmsmEmf_V) -> Delay/1
  VfSvc_iPmsmFlux_Wb/1 -> Subsystem1/4(VfSvc_iPmsmFlux_Wb)
  VfSvc_PreIq_A/1 -> Subsystem1/3(VfSvc_PreIq_A)
  Subsystem1/2(VfSvc_AxsiQeSpeedEst_rads) -> VfSvc_AxsiQeSpeedEst_rads/1
  Delay/1 -> Subsystem/7(VfSvc_iPmsmPreEmf_V)

== system MotorIPMSVC/SVC/iPmsmSvcParamCalc ==
  VfSvc_PWMFreq_Hz : Inport
  VfSvc_iPmsmLd_H : Inport  Port=2
  VfSvc_iPmsmLq_H : Inport  Port=3
  Product : Product
  Product1 : Product
  VfSvc_TpwmDivLd_H : Outport
  VfSvc_TpwmDivLq_H : Outport  Port=2
  wires:
  VfSvc_iPmsmLq_H/1 -> Product1/1
  Product1/1 -> VfSvc_TpwmDivLq_H/1
  VfSvc_PWMFreq_Hz/1 -> Product1/2, Product/1
  Product/1 -> VfSvc_TpwmDivLd_H/1
  VfSvc_iPmsmLd_H/1 -> Product/2

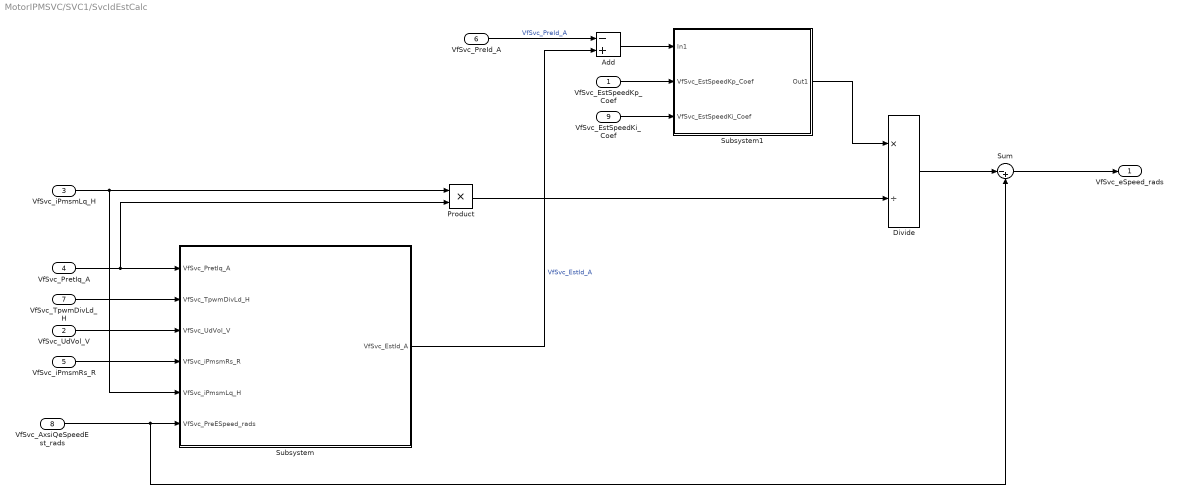
== system MotorIPMSVC/SVC1/SvcIdEstCalc ==
  VfSvc_EstSpeedKp_Coef : Inport
  VfSvc_UdVol_V : Inport  Port=2
  VfSvc_iPmsmLq_H : Inport  Port=3
  VfSvc_PretIq_A : Inport  Port=4
  VfSvc_iPmsmRs_R : Inport  Port=5
  VfSvc_PreId_A : Inport  Port=6
  VfSvc_TpwmDivLd_H : Inport  Port=7
  VfSvc_AxsiQeSpeedEst_rads : Inport  Port=8
  VfSvc_EstSpeedKi_Coef : Inport  Port=9
  Add : Sum  Inputs=-+
  Divide : Product  Inputs=*/
  Product : Product
  Subsystem : Subsystem
  Subsystem1 : Subsystem
  Sum : Sum  Inputs=|-+
  VfSvc_eSpeed_rads : Outport
  wires:
  VfSvc_TpwmDivLd_H/1 -> Subsystem/2(VfSvc_TpwmDivLd_H)
  VfSvc_UdVol_V/1 -> Subsystem/3(VfSvc_UdVol_V)
  VfSvc_PretIq_A/1 -> Product/2, Subsystem/1(VfSvc_PretIq_A)
  VfSvc_iPmsmRs_R/1 -> Subsystem/4(VfSvc_iPmsmRs_R)
  VfSvc_iPmsmLq_H/1 -> Product/1, Subsystem/5(VfSvc_iPmsmLq_H)
  Subsystem/1(VfSvc_EstId_A) -> Add/2  "VfSvc_EstId_A"
  VfSvc_PreId_A/1 -> Add/1  "VfSvc_PreId_A"
  Divide/1 -> Sum/1
  VfSvc_AxsiQeSpeedEst_rads/1 -> Sum/2, Subsystem/6(VfSvc_PreESpeed_rads)
  Sum/1 -> VfSvc_eSpeed_rads/1
  Product/1 -> Divide/2
  Add/1 -> Subsystem1/1(In1)
  VfSvc_EstSpeedKp_Coef/1 -> Subsystem1/2(VfSvc_EstSpeedKp_Coef)
  VfSvc_EstSpeedKi_Coef/1 -> Subsystem1/3(VfSvc_EstSpeedKi_Coef)
  Subsystem1/1(Out1) -> Divide/1

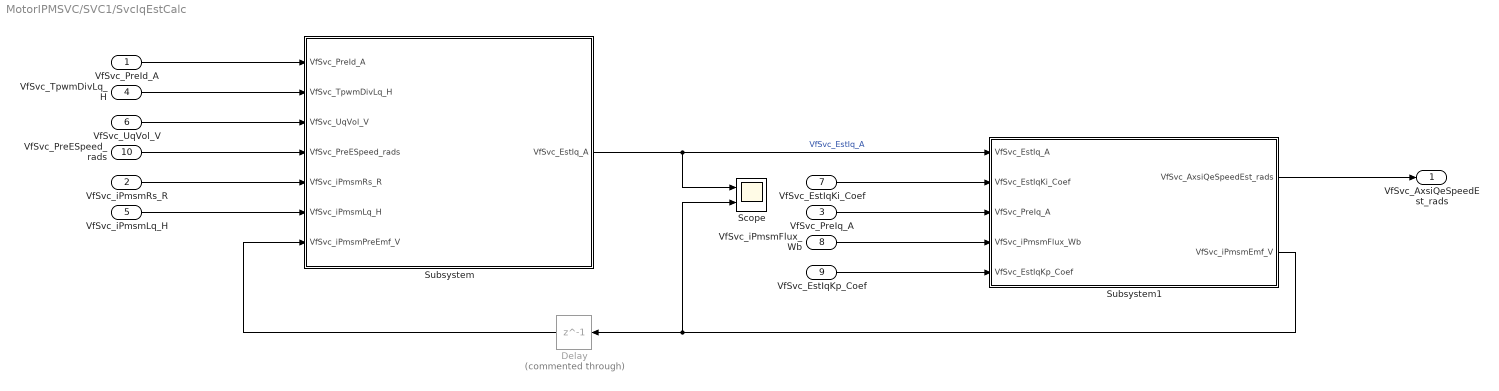
== system MotorIPMSVC/SVC1/SvcIqEstCalc ==
  VfSvc_PreId_A : Inport
  VfSvc_iPmsmRs_R : Inport  Port=2
  VfSvc_PreIq_A : Inport  Port=3
  VfSvc_TpwmDivLq_H : Inport  Port=4
  VfSvc_iPmsmLq_H : Inport  Port=5
  VfSvc_UqVol_V : Inport  Port=6
  VfSvc_EstIqKi_Coef : Inport  Port=7
  VfSvc_iPmsmFlux_Wb : Inport  Port=8
  VfSvc_EstIqKp_Coef : Inport  Port=9
  VfSvc_PreESpeed_rads : Inport  Port=10
  Delay : Delay  Commented=through  DelayLength=1
  Scope : Scope  NumInputPorts=2
  Subsystem : Subsystem
  Subsystem1 : Subsystem
  VfSvc_AxsiQeSpeedEst_rads : Outport
  wires:
  VfSvc_PreId_A/1 -> Subsystem/1(VfSvc_PreId_A)
  VfSvc_TpwmDivLq_H/1 -> Subsystem/2(VfSvc_TpwmDivLq_H)
  VfSvc_UqVol_V/1 -> Subsystem/3(VfSvc_UqVol_V)
  VfSvc_PreESpeed_rads/1 -> Subsystem/4(VfSvc_PreESpeed_rads)
  VfSvc_iPmsmRs_R/1 -> Subsystem/5(VfSvc_iPmsmRs_R)
  VfSvc_iPmsmLq_H/1 -> Subsystem/6(VfSvc_iPmsmLq_H)
  Subsystem/1(VfSvc_EstIq_A) -> Scope/1, Subsystem1/1(VfSvc_EstIq_A)  "VfSvc_EstIq_A"
  VfSvc_EstIqKi_Coef/1 -> Subsystem1/2(VfSvc_EstIqKi_Coef)
  VfSvc_iPmsmFlux_Wb/1 -> Subsystem1/4(VfSvc_iPmsmFlux_Wb)
  VfSvc_PreIq_A/1 -> Subsystem1/3(VfSvc_PreIq_A)
  Subsystem1/1(VfSvc_AxsiQeSpeedEst_rads) -> VfSvc_AxsiQeSpeedEst_rads/1
  VfSvc_EstIqKp_Coef/1 -> Subsystem1/5(VfSvc_EstIqKp_Coef)
  Subsystem1/2(VfSvc_iPmsmEmf_V) -> Scope/2, Delay/1
  Delay/1 -> Subsystem/7(VfSvc_iPmsmPreEmf_V)

== system MotorIPMSVC/SVC1/iPmsmSvcParamCalc ==
  VfSvc_PWMFreq_Hz : Inport
  VfSvc_iPmsmLd_H : Inport  Port=2
  VfSvc_iPmsmLq_H : Inport  Port=3
  Product : Product
  Product1 : Product
  VfSvc_TpwmDivLd_H : Outport
  VfSvc_TpwmDivLq_H : Outport  Port=2
  wires:
  VfSvc_iPmsmLq_H/1 -> Product1/1
  Product1/1 -> VfSvc_TpwmDivLq_H/1
  VfSvc_PWMFreq_Hz/1 -> Product1/2, Product/1
  Product/1 -> VfSvc_TpwmDivLd_H/1
  VfSvc_iPmsmLd_H/1 -> Product/2

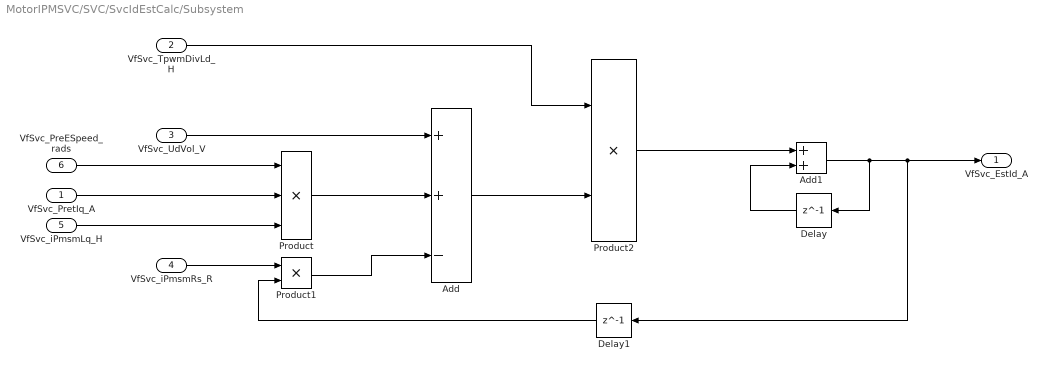
== system MotorIPMSVC/SVC/SvcIdEstCalc/Subsystem ==
  VfSvc_PretIq_A : Inport
  VfSvc_TpwmDivLd_H : Inport  Port=2
  VfSvc_UdVol_V : Inport  Port=3
  VfSvc_iPmsmRs_R : Inport  Port=4
  VfSvc_iPmsmLq_H : Inport  Port=5
  VfSvc_PreESpeed_rads : Inport  Port=6
  Add : Sum  Inputs=++-
  Add1 : Sum
  Delay : Delay  DelayLength=1
  Delay1 : Delay  DelayLength=1
  Product : Product  Inputs=3
  Product1 : Product
  Product2 : Product
  VfSvc_EstId_A : Outport
  wires:
  VfSvc_UdVol_V/1 -> Add/1
  VfSvc_PreESpeed_rads/1 -> Product/1
  VfSvc_TpwmDivLd_H/1 -> Product2/1
  VfSvc_PretIq_A/1 -> Product/2
  VfSvc_iPmsmRs_R/1 -> Product1/1
  Add1/1 -> Delay/1, VfSvc_EstId_A/1, Delay1/1
  Product/1 -> Add/2
  Product2/1 -> Add1/1
  Product1/1 -> Add/3
  Add/1 -> Product2/2
  Delay/1 -> Add1/2
  VfSvc_iPmsmLq_H/1 -> Product/3
  Delay1/1 -> Product1/2

== system MotorIPMSVC/SVC/SvcIqEstCalc/Subsystem ==
  VfSvc_PreId_A : Inport
  VfSvc_TpwmDivLq_H : Inport  Port=2
  VfSvc_UqVol_V : Inport  Port=3
  VfSvc_PreESpeed_rads : Inport  Port=4
  VfSvc_iPmsmRs_R : Inport  Port=5
  VfSvc_iPmsmLq_H : Inport  Port=6
  VfSvc_iPmsmPreEmf_V : Inport  Port=7
  Subsystem : Subsystem
  VfSvc_EstIq_A : Outport
  wires:
  VfSvc_PreId_A/1 -> Subsystem/1(VfSvc_PreId_A)
  VfSvc_TpwmDivLq_H/1 -> Subsystem/2(VfSvc_TpwmDivLq_H)
  VfSvc_UqVol_V/1 -> Subsystem/3(VfSvc_UqVol_V)
  VfSvc_PreESpeed_rads/1 -> Subsystem/4(VfSvc_PreESpeed_rads)
  VfSvc_iPmsmRs_R/1 -> Subsystem/5(VfSvc_iPmsmRs_R)
  VfSvc_iPmsmLq_H/1 -> Subsystem/6(VfSvc_iPmsmLq_H)
  VfSvc_iPmsmPreEmf_V/1 -> Subsystem/7(VfSvc_iPmsmPreEmf_V)
  Subsystem/1(VfSvc_EstIq_A) -> VfSvc_EstIq_A/1

== system MotorIPMSVC/SVC/SvcIqEstCalc/Subsystem1 ==
  VfSvc_EstIq_A : Inport
  VfSvc_EstIqKi_Coef : Inport  Port=2
  VfSvc_PreIq_A : Inport  Port=3
  VfSvc_iPmsmFlux_Wb : Inport  Port=4
  Add : Sum  Inputs=-+
  Add1 : Sum
  Delay : Delay  DelayLength=1
  Divide : Product  Inputs=*/
  Product : Product
  VfSvc_iPmsmEmf_V : Outport
  VfSvc_AxsiQeSpeedEst_rads : Outport  Port=2
  wires:
  Product/1 -> Add1/1
  VfSvc_EstIqKi_Coef/1 -> Product/1
  VfSvc_PreIq_A/1 -> Add/1
  Add1/1 -> Divide/1, VfSvc_iPmsmEmf_V/1, Delay/1
  Add/1 -> Product/2
  Delay/1 -> Add1/2
  VfSvc_EstIq_A/1 -> Add/2
  VfSvc_iPmsmFlux_Wb/1 -> Divide/2
  Divide/1 -> VfSvc_AxsiQeSpeedEst_rads/1

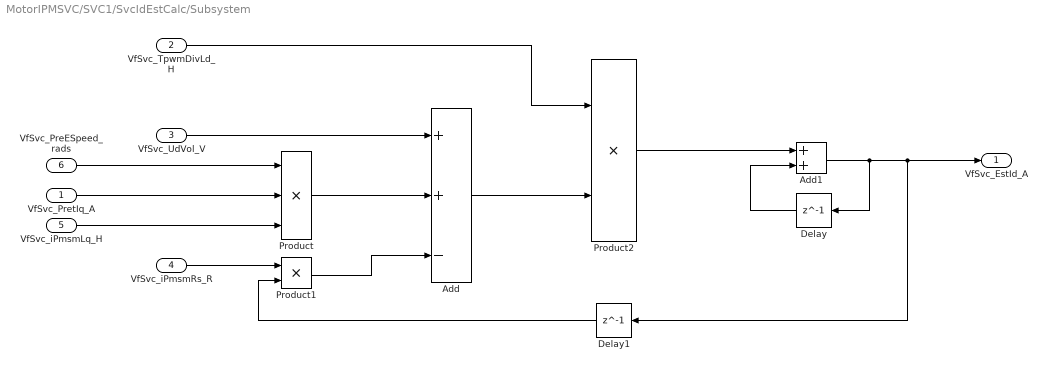
== system MotorIPMSVC/SVC1/SvcIdEstCalc/Subsystem ==
  VfSvc_PretIq_A : Inport
  VfSvc_TpwmDivLd_H : Inport  Port=2
  VfSvc_UdVol_V : Inport  Port=3
  VfSvc_iPmsmRs_R : Inport  Port=4
  VfSvc_iPmsmLq_H : Inport  Port=5
  VfSvc_PreESpeed_rads : Inport  Port=6
  Add : Sum  Inputs=++-
  Add1 : Sum
  Delay : Delay  DelayLength=1
  Delay1 : Delay  DelayLength=1
  Product : Product  Inputs=3
  Product1 : Product
  Product2 : Product
  VfSvc_EstId_A : Outport
  wires:
  VfSvc_UdVol_V/1 -> Add/1
  VfSvc_PreESpeed_rads/1 -> Product/1
  VfSvc_TpwmDivLd_H/1 -> Product2/1
  VfSvc_PretIq_A/1 -> Product/2
  VfSvc_iPmsmRs_R/1 -> Product1/1
  Add1/1 -> Delay/1, VfSvc_EstId_A/1, Delay1/1
  Product/1 -> Add/2
  Product2/1 -> Add1/1
  Product1/1 -> Add/3
  Add/1 -> Product2/2
  Delay/1 -> Add1/2
  VfSvc_iPmsmLq_H/1 -> Product/3
  Delay1/1 -> Product1/2

== system MotorIPMSVC/SVC1/SvcIdEstCalc/Subsystem1 ==
  In1 : Inport
  VfSvc_EstSpeedKp_Coef : Inport  Port=2
  VfSvc_EstSpeedKi_Coef : Inport  Port=3
  Add1 : Sum
  Add2 : Sum
  Delay : Delay  DelayLength=1
  Product1 : Product
  Product2 : Product
  Out1 : Outport
  wires:
  Delay/1 -> Add1/2
  Add1/1 -> Add2/2, Delay/1
  In1/1 -> Product1/1, Product2/1
  Product2/1 -> Add1/1
  VfSvc_EstSpeedKi_Coef/1 -> Product2/2
  VfSvc_EstSpeedKp_Coef/1 -> Product1/2
  Product1/1 -> Add2/1
  Add2/1 -> Out1/1

== system MotorIPMSVC/SVC1/SvcIqEstCalc/Subsystem ==
  VfSvc_PreId_A : Inport
  VfSvc_TpwmDivLq_H : Inport  Port=2
  VfSvc_UqVol_V : Inport  Port=3
  VfSvc_PreESpeed_rads : Inport  Port=4
  VfSvc_iPmsmRs_R : Inport  Port=5
  VfSvc_iPmsmLq_H : Inport  Port=6
  VfSvc_iPmsmPreEmf_V : Inport  Port=7
  Subsystem : Subsystem
  VfSvc_EstIq_A : Outport
  wires:
  VfSvc_PreId_A/1 -> Subsystem/1(VfSvc_PreId_A)
  VfSvc_TpwmDivLq_H/1 -> Subsystem/2(VfSvc_TpwmDivLq_H)
  VfSvc_UqVol_V/1 -> Subsystem/3(VfSvc_UqVol_V)
  VfSvc_PreESpeed_rads/1 -> Subsystem/4(VfSvc_PreESpeed_rads)
  VfSvc_iPmsmRs_R/1 -> Subsystem/5(VfSvc_iPmsmRs_R)
  VfSvc_iPmsmLq_H/1 -> Subsystem/6(VfSvc_iPmsmLq_H)
  VfSvc_iPmsmPreEmf_V/1 -> Subsystem/7(VfSvc_iPmsmPreEmf_V)
  Subsystem/1(VfSvc_EstIq_A) -> VfSvc_EstIq_A/1

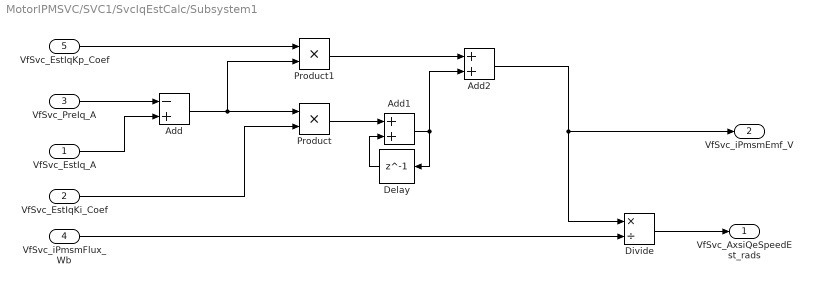
== system MotorIPMSVC/SVC1/SvcIqEstCalc/Subsystem1 ==
  VfSvc_EstIq_A : Inport
  VfSvc_EstIqKi_Coef : Inport  Port=2
  VfSvc_PreIq_A : Inport  Port=3
  VfSvc_iPmsmFlux_Wb : Inport  Port=4
  VfSvc_EstIqKp_Coef : Inport  Port=5
  Add : Sum  Inputs=-+
  Add1 : Sum
  Add2 : Sum
  Delay : Delay  DelayLength=1
  Divide : Product  Inputs=*/
  Product : Product
  Product1 : Product
  VfSvc_AxsiQeSpeedEst_rads : Outport
  VfSvc_iPmsmEmf_V : Outport  Port=2
  wires:
  Product/1 -> Add1/1
  VfSvc_EstIqKi_Coef/1 -> Product/2
  VfSvc_PreIq_A/1 -> Add/1
  Add1/1 -> Add2/2, Delay/1
  Add/1 -> Product/1, Product1/2
  Delay/1 -> Add1/2
  VfSvc_EstIq_A/1 -> Add/2
  VfSvc_iPmsmFlux_Wb/1 -> Divide/2
  Divide/1 -> VfSvc_AxsiQeSpeedEst_rads/1
  VfSvc_EstIqKp_Coef/1 -> Product1/1
  Product1/1 -> Add2/1
  Add2/1 -> VfSvc_iPmsmEmf_V/1, Divide/1

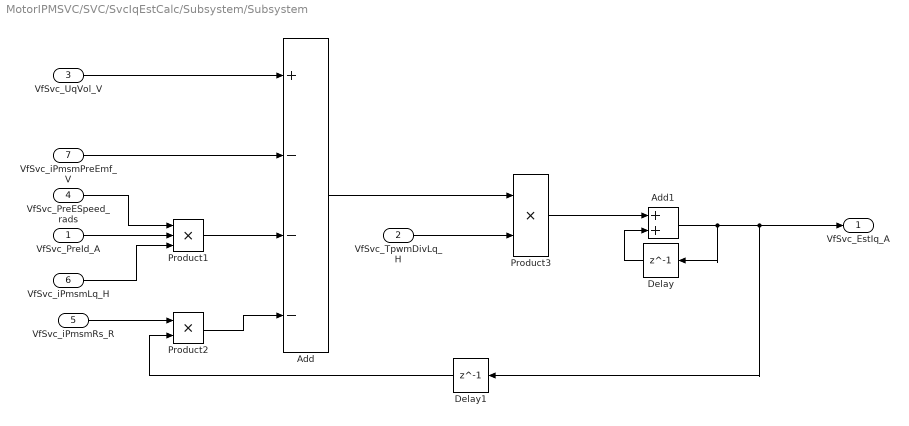
== system MotorIPMSVC/SVC/SvcIqEstCalc/Subsystem/Subsystem ==
  VfSvc_PreId_A : Inport
  VfSvc_TpwmDivLq_H : Inport  Port=2
  VfSvc_UqVol_V : Inport  Port=3
  VfSvc_PreESpeed_rads : Inport  Port=4
  VfSvc_iPmsmRs_R : Inport  Port=5
  VfSvc_iPmsmLq_H : Inport  Port=6
  VfSvc_iPmsmPreEmf_V : Inport  Port=7
  Add : Sum  Inputs=+---
  Add1 : Sum
  Delay : Delay  DelayLength=1
  Delay1 : Delay  DelayLength=1
  Product1 : Product  Inputs=3
  Product2 : Product
  Product3 : Product
  VfSvc_EstIq_A : Outport
  wires:
  VfSvc_iPmsmRs_R/1 -> Product2/1
  Add1/1 -> Delay/1, VfSvc_EstIq_A/1, Delay1/1
  Add/1 -> Product3/1
  VfSvc_iPmsmLq_H/1 -> Product1/3
  VfSvc_iPmsmPreEmf_V/1 -> Add/2
  Delay/1 -> Add1/2
  VfSvc_TpwmDivLq_H/1 -> Product3/2
  VfSvc_UqVol_V/1 -> Add/1
  Product3/1 -> Add1/1
  Product1/1 -> Add/3
  VfSvc_PreId_A/1 -> Product1/2
  VfSvc_PreESpeed_rads/1 -> Product1/1
  Product2/1 -> Add/4
  Delay1/1 -> Product2/2

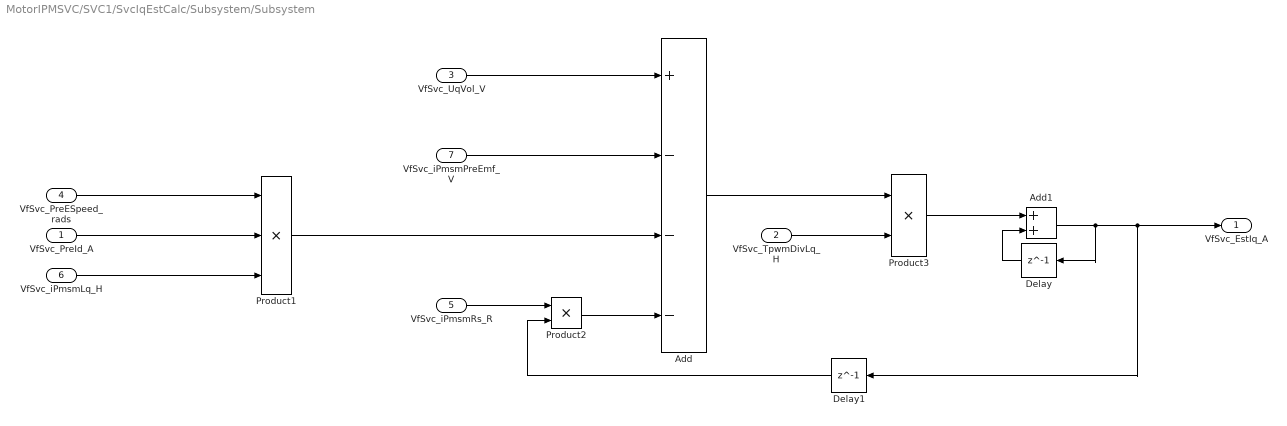
== system MotorIPMSVC/SVC1/SvcIqEstCalc/Subsystem/Subsystem ==
  VfSvc_PreId_A : Inport
  VfSvc_TpwmDivLq_H : Inport  Port=2
  VfSvc_UqVol_V : Inport  Port=3
  VfSvc_PreESpeed_rads : Inport  Port=4
  VfSvc_iPmsmRs_R : Inport  Port=5
  VfSvc_iPmsmLq_H : Inport  Port=6
  VfSvc_iPmsmPreEmf_V : Inport  Port=7
  Add : Sum  Inputs=+---
  Add1 : Sum
  Delay : Delay  DelayLength=1
  Delay1 : Delay  DelayLength=1
  Product1 : Product  Inputs=3
  Product2 : Product
  Product3 : Product
  VfSvc_EstIq_A : Outport
  wires:
  VfSvc_iPmsmRs_R/1 -> Product2/1
  Add1/1 -> Delay/1, VfSvc_EstIq_A/1, Delay1/1
  Add/1 -> Product3/1
  VfSvc_iPmsmLq_H/1 -> Product1/3
  VfSvc_iPmsmPreEmf_V/1 -> Add/2
  Delay/1 -> Add1/2
  VfSvc_TpwmDivLq_H/1 -> Product3/2
  VfSvc_UqVol_V/1 -> Add/1
  Product3/1 -> Add1/1
  Product1/1 -> Add/3
  VfSvc_PreId_A/1 -> Product1/2
  VfSvc_PreESpeed_rads/1 -> Product1/1
  Product2/1 -> Add/4
  Delay1/1 -> Product2/2
